simulink model "Test_qrate"  (R2017a)
settings: Solver=VariableStepAuto  StartTime=0.0  StopTime=20  RelTol=1e-3  EnableMultiTasking=on
InitFcn:
  | clear all;
  | load('Parameters.mat');
undefined symbols (not defined in the file): A_AC_LONG_SS, B_AC_LONG_SS, C_AC_LONG_SS, D_AC_LONG_SS, trim_control_hi
libraries: simulink x1
settings Model: Creator=Y Nie  LastModifiedBy=aelabuser
settings DataIOCC: SaveFormat=Array  SignalLoggingSaveFormat=ModelDataLogs  SaveOutput=off  SignalLogging=off  DSMLogging=off  TimeSaveName=TestTime
settings OptimizationCC: ExpressionDepthLimit=2147483647  LifeSpan=inf
settings DebuggingCC: UnderspecifiedInitializationDetection=Classic  MergeDetectMultiDrivingBlocksExec=none  FcnCallInpInsideContextMsg=warning  StateNameClashWarn=warning  SFUnexpectedBacktrackingDiag=warning  SFNoUnconditionalDefaultTransitionDiag=warning  SFExecutionAtInitializationDiag=none
settings HardwareCC: ProdBitPerPointer=32  ProdBitPerSizeT=32  ProdBitPerPtrDiffT=32  ProdLargestAtomicFloat=None  ProdIntDivRoundTo=Undefined  ProdEndianess=Unspecified  ProdWordSize=32  ProdHWDeviceType=32-bit Generic
settings ModelReferenceCC: PropagateSignalLabelsOutOfModel=off
settings GRTTargetCC: TargetLangStandard=C89/C90 (ANSI)  GeneratePreprocessorConditionals=Disable all  CombineOutputUpdateFcns=off  GRTInterface=on
settings ConfigComp: CovMetricSettings=dw  CovHtmlReporting=on  CovSaveCumulativeToWorkspaceVar=on  CovSaveSingleToWorkspaceVar=on  CovExternalEMLEnable=off

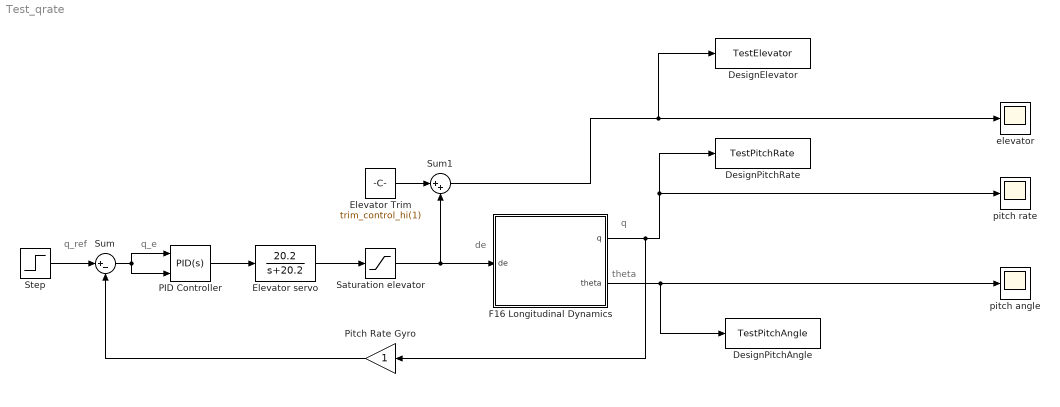
== system Test_qrate ==
  note: q
  note: theta
  note: q_e
  note: q_ref
  note: de
  DesignElevator : ToWorkspace  VariableName=TestElevator  SampleTime=-1
  DesignPitchAngle : ToWorkspace  VariableName=TestPitchAngle  SampleTime=-1
  DesignPitchRate : ToWorkspace  VariableName=TestPitchRate  SampleTime=-1
  Elevator Trim : Constant  Value=trim_control_hi(1)
  Elevator servo : TransferFcn  Numerator=[20.2]  Denominator=[1 20.2]
  F16 Longitudinal Dynamics : Subsystem
      mask Display: image(imread('f16thumb.jpg'))
  PID Controller : simulink/Continuous/PID Controller  Controller=PID  TimeDomain=Continuous-time  SampleTime=-1  IntegratorMethod=Forward Euler  FilterMethod=Forward Euler  Form=Parallel  UseFilter=on  ControllerParametersSource=internal  P=0  I=0  D=0  N=100  InitialConditionSource=internal  InitialConditionForIntegrator=0  InitialConditionForFilter=0  ExternalReset=either  LimitOutput=off  UpperSaturationLimit=inf  LowerSaturationLimit=-inf  LinearizeAsGain=on  AntiWindupMode=none  Kb=1  TrackingMode=off  Kt=1  PParamMin=[]  PParamMax=[]  IParamMin=[]  IParamMax=[]  DParamMin=[]  DParamMax=[]  NParamMin=[]  NParamMax=[]  KbParamMin=[]  KbParamMax=[]  KtParamMin=[]  KtParamMax=[]  POutMin=[]  POutMax=[]  IOutMin=[]  IOutMax=[]  DOutMin=[]  DOutMax=[]  NOutMin=[]  NOutMax=[]  KbOutMin=[]  KbOutMax=[]  KtOutMin=[]  KtOutMax=[]  IntegratorOutMin=[]  IntegratorOutMax=[]  FilterOutMin=[]  FilterOutMax=[]  SumOutMin=[]  SumOutMax=[]  SumI1OutMin=[]  SumI1OutMax=[]  SumI2OutMin=[]  SumI2OutMax=[]  SumI3OutMin=[]  SumI3OutMax=[]  SumDOutMin=[]  SumDOutMax=[]  SaturationOutMin=[]  SaturationOutMax=[]  IntegratorContinuousStateAttributes=''  IntegratorStateMustResolveToSignalObject=off  IntegratorRTWStateStorageClass=Auto  FilterContinuousStateAttributes=''  FilterStateMustResolveToSignalObject=off  FilterRTWStateStorageClass=Auto  DifferentiatorICPrevScaledInput=0  DifferentiatorOutMin=[]  DifferentiatorOutMax=[]  InitialConditionSetting=State (most efficient)
  Pitch Rate Gyro : Gain
  Saturation elevator : Saturate  UpperLimit=25-trim_control_hi(1)  LowerLimit=-25-trim_control_hi(1)
  Step : Step  Time=10  Before=1  After=0  SampleTime=0
  Sum : Sum  Inputs=|+-
  Sum1 : Sum  Inputs=|++
  elevator : Scope
  pitch angle : Scope
  pitch rate : Scope
  wires:
  Sum1/1 -> elevator/1, DesignElevator/1
  Elevator Trim/1 -> Sum1/1
  F16 Longitudinal Dynamics/2(theta) -> pitch angle/1, DesignPitchAngle/1
  PID Controller/1 -> Elevator servo/1
  Pitch Rate Gyro/1 -> Sum/2
  Elevator servo/1 -> Saturation elevator/1
  Sum/1 -> PID Controller/2, PID Controller/1
  Saturation elevator/1 -> Sum1/2, F16 Longitudinal Dynamics/1(de)
  F16 Longitudinal Dynamics/1(q) -> Pitch Rate Gyro/1, DesignPitchRate/1, pitch rate/1
  Step/1 -> Sum/1

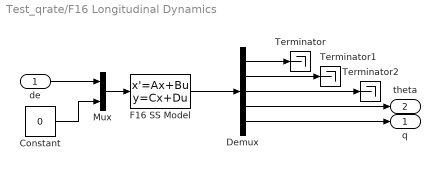
== system Test_qrate/F16 Longitudinal Dynamics ==
  de : Inport
  Constant : Constant  Value=0
  Demux : Demux  Outputs=5
  F16 SS Model : StateSpace  A=A_AC_LONG_SS  B=B_AC_LONG_SS  C=C_AC_LONG_SS  D=D_AC_LONG_SS  X0=0
  Mux : Mux  Inputs=2
  Terminator : Terminator
  Terminator1 : Terminator
  Terminator2 : Terminator
  q : Outport
  theta : Outport  Port=2
  wires:
  Mux/1 -> F16 SS Model/1
  de/1 -> Mux/1
  Constant/1 -> Mux/2
  F16 SS Model/1 -> Demux/1
  Demux/5 -> q/1
  Demux/4 -> theta/1
  Demux/1 -> Terminator/1
  Demux/2 -> Terminator1/1
  Demux/3 -> Terminator2/1
